simulink library "MOVH"  (R2016a)
settings: Solver=ode45  StartTime=0.0  StopTime=10.0  RelTol=1e-3
undefined symbols (not defined in the file): ALLOWED_ERROR_VALUE, BACKWARD, CCW, CW, FORWARD, MOVE_TURN_LEFT, MOVE_TURN_RIGHT, MOVE_U_TURN, MOVE_U_TURN_LEFT, MOVE_U_TURN_RIGHT, NO_ERROR, ROB_EAST, ROB_NORTH, ROB_SOUTH, ROB_WEST, STOP
libraries: simulink x2
settings Model: Creator=oelkawok  LastModifiedBy=oelkawok
settings DataIOCC: LimitDataPoints=on
settings DebuggingCC: AllowSymbolicDim=off

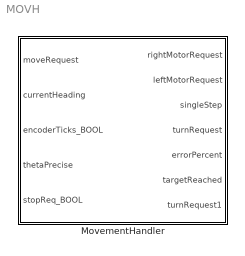
== system MOVH ==
  MovementHandler : Subsystem

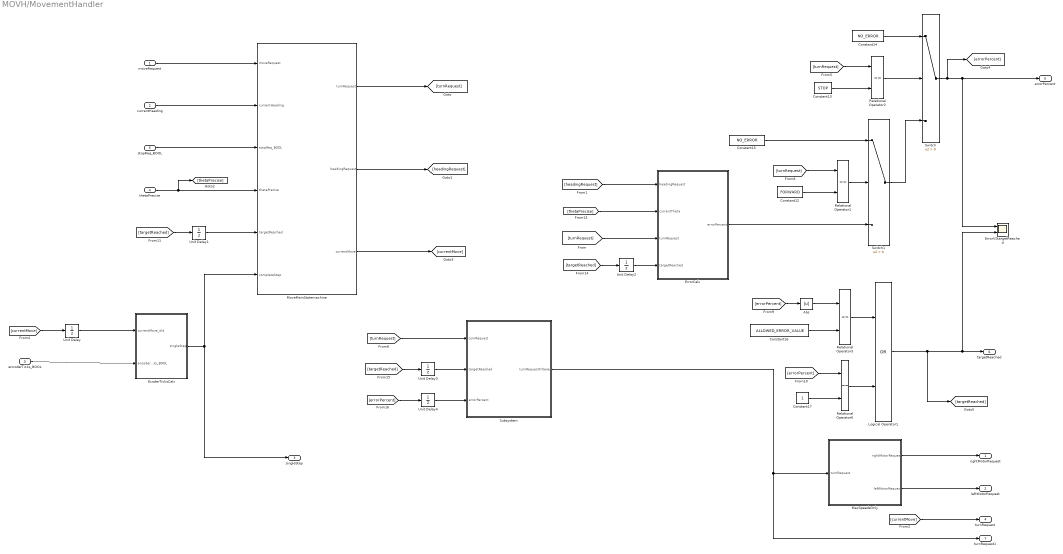
== system MOVH/MovementHandler ==
  moveRequest : Inport
  currentHeading : Inport  Port=2
  encoderTicks_BOOL : Inport  Port=3  PortDimensions=1
  thetaPrecise : Inport  Port=4  PortDimensions=1
  stopReq_BOOL : Inport  Port=5  PortDimensions=1
  Abs : Abs
  Constant12 : Constant  Value=FORWARD
  Constant13 : Constant  Value=STOP
  Constant14 : Constant  Value=NO_ERROR
  Constant15 : Constant  Value=NO_ERROR
  Constant16 : Constant  Value=ALLOWED_ERROR_VALUE
  Constant17 : Constant
  EcoderTicksCalc : Subsystem
  ErrorCalc : Subsystem
  ErrorVStargetReached : Scope  NumInputPorts=2
  Logical Operator1 : Logic  Operator=OR  AllPortsSameDT=off  OutDataTypeStr=boolean
  MaxSpeedsOnly : Subsystem
  MoveMainStatemachine : Subsystem
  Relational Operator1 : RelationalOperator  Operator===  OutDataTypeStr=boolean
  Relational Operator2 : RelationalOperator  Operator===  OutDataTypeStr=boolean
  Relational Operator3 : RelationalOperator  Operator=<=  OutDataTypeStr=boolean
  Relational Operator6 : RelationalOperator  Operator===  OutDataTypeStr=boolean
  Subsystem : Subsystem
  Switch : Switch  Criteria=u2 > Threshold
  Switch1 : Switch  Criteria=u2 > Threshold
  Unit Delay : UnitDelay  InitialCondition=STOP  SampleTime=-1
      settings: AttributesFormatString=%<InitialCondition>
  Unit Delay{1..4} (4 alike) : UnitDelay  InitialCondition=NO_ERROR  SampleTime=-1
      settings: AttributesFormatString=%<InitialCondition>
  rightMotorRequest : Outport
  leftMotorRequest : Outport  Port=2
  singleStep : Outport  Port=3
  turnRequest : Outport  Port=4
  errorPercent : Outport  Port=5  OutputWhenDisabled=reset  InitialOutput=0
  targetReached : Outport  Port=6  OutputWhenDisabled=reset  InitialOutput=0
  turnRequest1 : Outport  Port=7
  wires:
  encoderTicks_BOOL/1 -> EcoderTicksCalc/2(encoderTicks_BOOL)
  EcoderTicksCalc/1(singleStep) -> singleStep/1, MoveMainStatemachine/6(completeStep)
  Constant15/1 -> Switch1/1
  Subsystem/1(turnRequestFiltered) -> turnRequest1/1, MaxSpeedsOnly/1(turnRequest)
  Abs/1 -> Relational Operator3/1
  [errorPercent] -> Unit Delay4/1
  Unit Delay4/1 -> Subsystem/3(errorPercent)
  Unit Delay3/1 -> Subsystem/2(targetReached)
  [targetReached] -> Unit Delay3/1
  Unit Delay2/1 -> ErrorCalc/4(targetReached)
  [targetReached] -> Unit Delay2/1
  Logical Operator1/1 -> targetReached/1, ErrorVStargetReached/2, [targetReached]
  Relational Operator6/1 -> Logical Operator1/2
  Relational Operator3/1 -> Logical Operator1/1
  Constant17/1 -> Relational Operator6/2
  [errorPercent] -> Relational Operator6/1
  Constant16/1 -> Relational Operator3/2
  [errorPercent] -> Abs/1
  Switch/1 -> errorPercent/1, ErrorVStargetReached/1, [errorPercent]
  ErrorCalc/1(errorPercent) -> Switch1/3
  Relational Operator1/1 -> Switch1/2
  [turnRequest] -> Relational Operator1/1
  Constant12/1 -> Relational Operator1/2
  Switch1/1 -> Switch/3
  Constant14/1 -> Switch/1
  Relational Operator2/1 -> Switch/2
  [turnRequest] -> Relational Operator2/1
  Constant13/1 -> Relational Operator2/2
  [currentMove] -> turnRequest/1
  [turnRequest] -> ErrorCalc/3(turnRequest)
  [headingRequest] -> ErrorCalc/1(headingRequest)
  [turnRequest] -> Subsystem/1(turnRequest)
  MaxSpeedsOnly/2(leftMotorRequest) -> leftMotorRequest/1
  MaxSpeedsOnly/1(rightMotorRequest) -> rightMotorRequest/1
  [currentMove] -> Unit Delay/1
  moveRequest/1 -> MoveMainStatemachine/1(moveRequest)
  stopReq_BOOL/1 -> MoveMainStatemachine/3(stopReq_BOOL)
  MoveMainStatemachine/1(turnRequest) -> [turnRequest]
  MoveMainStatemachine/2(headingRequest) -> [headingRequest]
  MoveMainStatemachine/3(currentMove) -> [currentMove]
  currentHeading/1 -> MoveMainStatemachine/2(currentHeading)
  thetaPrecise/1 -> [thetaPrecise], MoveMainStatemachine/4(thetaPrecise)
  [thetaPrecise] -> ErrorCalc/2(currentTheta)
  [targetReached] -> Unit Delay1/1
  Unit Delay1/1 -> MoveMainStatemachine/5(targetReached)
  Unit Delay/1 -> EcoderTicksCalc/1(currentMove_old)

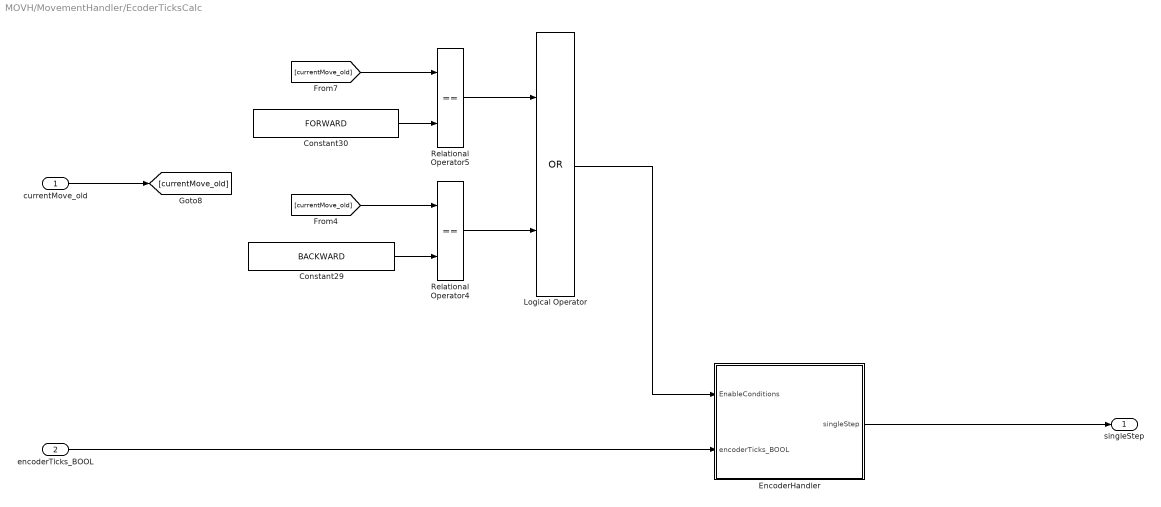
== system MOVH/MovementHandler/EcoderTicksCalc ==
  currentMove_old : Inport
  encoderTicks_BOOL : Inport  Port=2
  Constant29 : Constant  Value=BACKWARD
  Constant30 : Constant  Value=FORWARD
  EncoderHandler : Subsystem
  Logical Operator : Logic  Operator=OR  AllPortsSameDT=off  OutDataTypeStr=boolean
  Relational Operator4 : RelationalOperator  Operator===  OutDataTypeStr=boolean
  Relational Operator5 : RelationalOperator  Operator===  OutDataTypeStr=boolean
  singleStep : Outport
  wires:
  currentMove_old/1 -> [currentMove_old]
  EncoderHandler/1(singleStep) -> singleStep/1
  Relational Operator4/1 -> Logical Operator/2
  Relational Operator5/1 -> Logical Operator/1
  [currentMove_old] -> Relational Operator5/1
  Constant30/1 -> Relational Operator5/2
  [currentMove_old] -> Relational Operator4/1
  Logical Operator/1 -> EncoderHandler/1(EnableConditions)
  encoderTicks_BOOL/1 -> EncoderHandler/2(encoderTicks_BOOL)
  Constant29/1 -> Relational Operator4/2

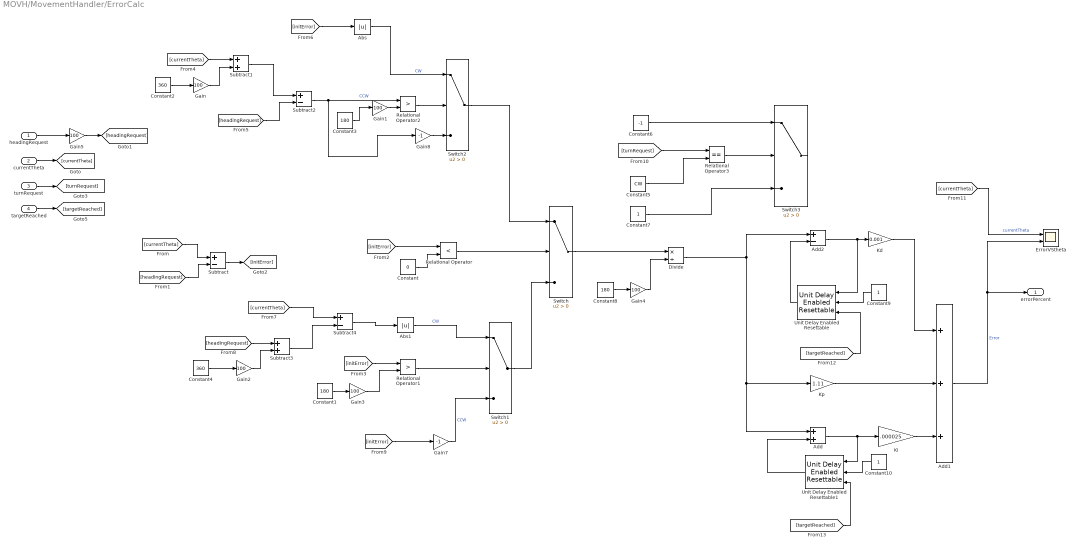
== system MOVH/MovementHandler/ErrorCalc ==
  headingRequest : Inport
  currentTheta : Inport  Port=2
  turnRequest : Inport  Port=3
  targetReached : Inport  Port=4
  Abs : Abs
  Abs1 : Abs
  Add : Sum
  Add1 : Sum  Inputs=+++
  Add2 : Sum  Inputs=+-
  Constant : Constant  Value=0
  Constant1 : Constant  Value=180
  Constant10 : Constant
  Constant2 : Constant  Value=360
  Constant3 : Constant  Value=180
  Constant4 : Constant  Value=360
  Constant5 : Constant  Value=CW
  Constant6 : Constant  Value=-1
  Constant7 : Constant
  Constant8 : Constant  Value=180
  Constant9 : Constant
  Divide : Product  Inputs=*/
  ErrorVStheta : Scope  NumInputPorts=2
  Gain{,1..5} (6 alike) : Gain  Gain=100
  Gain7 : Gain  Gain=-1
  Gain8 : Gain  Gain=-1
  Kd : Gain  Gain=0.001
  Ki : Gain  Gain=.000025
  Kp : Gain  Gain=1.11
  Relational Operator : RelationalOperator  Operator=<  OutDataTypeStr=boolean
  Relational Operator1 : RelationalOperator  Operator=>  OutDataTypeStr=boolean
  Relational Operator2 : RelationalOperator  Operator=>  OutDataTypeStr=boolean
  Relational Operator3 : RelationalOperator  Operator===  OutDataTypeStr=boolean
  Subtract : Sum  Inputs=+-
  Subtract1 : Sum
  Subtract2 : Sum  Inputs=+-
  Subtract3 : Sum
  Subtract4 : Sum  Inputs=+-
  Switch{,1..3} (4 alike) : Switch  Criteria=u2 > Threshold
  Unit Delay Enabled Resettable : simulink/Additional Math & Discrete/Additional Discrete/Unit Delay Enabled Resettable  vinit=0.0  tsamp=-1
  Unit Delay Enabled Resettable1 : simulink/Additional Math & Discrete/Additional Discrete/Unit Delay Enabled Resettable  vinit=0.0  tsamp=-1
  errorPercent : Outport  OutputWhenDisabled=reset  InitialOutput=0
  wires:
  Gain8/1 -> Switch2/3
  Gain7/1 -> Switch1/3  "CCW"
  [targetReached] -> Unit Delay Enabled Resettable1/3
  Constant10/1 -> Unit Delay Enabled Resettable1/2
  [targetReached] -> Unit Delay Enabled Resettable/3
  targetReached/1 -> [targetReached]
  Constant9/1 -> Unit Delay Enabled Resettable/2
  Gain5/1 -> [headingRequest]
  Gain4/1 -> Divide/2
  Gain3/1 -> Relational Operator1/2
  Gain2/1 -> Subtract3/2
  Gain1/1 -> Relational Operator2/2
  Gain/1 -> Subtract1/2
  [currentTheta] -> ErrorVStheta/1  "currentTheta"
  Add1/1 -> errorPercent/1, ErrorVStheta/2  "Error"
  Kp/1 -> Add1/2
  Kd/1 -> Add1/1
  Unit Delay Enabled Resettable/1 -> Add2/2
  Add2/1 -> Kd/1, Unit Delay Enabled Resettable/1
  Ki/1 -> Add1/3
  Unit Delay Enabled Resettable1/1 -> Add/2
  Add/1 -> Ki/1, Unit Delay Enabled Resettable1/1
  Divide/1 -> Add/1, Kp/1, Add2/1
  Constant/1 -> Relational Operator/2
  Relational Operator/1 -> Switch/2
  Relational Operator1/1 -> Switch1/2
  Constant1/1 -> Gain3/1
  Switch1/1 -> Switch/3
  headingRequest/1 -> Gain5/1
  currentTheta/1 -> [currentTheta]
  [headingRequest] -> Subtract/2
  [currentTheta] -> Subtract/1
  Subtract/1 -> [initError]
  [initError] -> Relational Operator/1
  [initError] -> Relational Operator1/1
  [currentTheta] -> Subtract1/1
  Constant2/1 -> Gain/1
  Subtract1/1 -> Subtract2/1
  [headingRequest] -> Subtract2/2
  Constant3/1 -> Gain1/1
  Subtract2/1 -> Relational Operator2/1, Gain8/1  "CCW"
  Relational Operator2/1 -> Switch2/2
  Switch2/1 -> Switch/1
  [initError] -> Abs/1
  Abs/1 -> Switch2/1  "CW"
  Constant4/1 -> Gain2/1
  [headingRequest] -> Subtract3/1
  [currentTheta] -> Subtract4/1
  Subtract3/1 -> Subtract4/2
  Subtract4/1 -> Abs1/1
  Abs1/1 -> Switch1/1  "CW"
  [initError] -> Gain7/1
  turnRequest/1 -> [turnRequest]
  [turnRequest] -> Relational Operator3/1
  Constant5/1 -> Relational Operator3/2
  Relational Operator3/1 -> Switch3/2
  Constant6/1 -> Switch3/1
  Constant7/1 -> Switch3/3
  Switch/1 -> Divide/1
  Constant8/1 -> Gain4/1

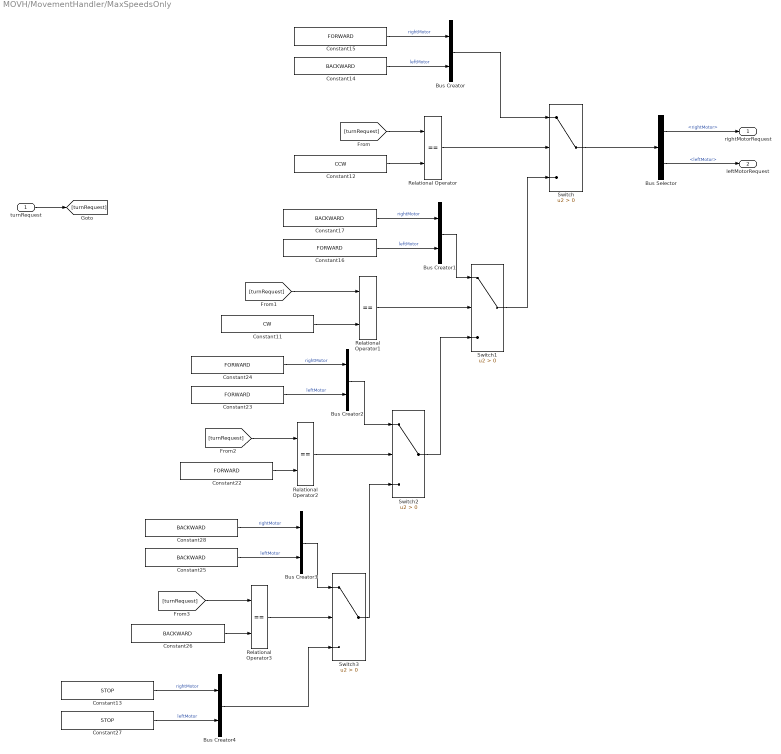
== system MOVH/MovementHandler/MaxSpeedsOnly ==
  turnRequest : Inport
  Bus Creator{,1..4} (5 alike) : BusCreator  Inputs=2
  Bus Selector : BusSelector  OutputSignals=rightMotor,leftMotor
  Constant11 : Constant  Value=CW
  Constant12 : Constant  Value=CCW
  Constant13 : Constant  Value=STOP
  Constant{14,17,25..26,28} (5 alike) : Constant  Value=BACKWARD
  Constant{15..16,22..24} (5 alike) : Constant  Value=FORWARD
  Constant27 : Constant  Value=STOP
  Relational Operator{,1..3} (4 alike) : RelationalOperator  Operator===  OutDataTypeStr=boolean
  Switch{,1..3} (4 alike) : Switch  Criteria=u2 > Threshold
  rightMotorRequest : Outport
  leftMotorRequest : Outport  Port=2
  wires:
  turnRequest/1 -> [turnRequest]
  Constant13/1 -> Bus Creator4/1  "rightMotor"
  Constant23/1 -> Bus Creator2/2  "leftMotor"
  Bus Creator3/1 -> Switch3/1
  Constant27/1 -> Bus Creator4/2  "leftMotor"
  Switch3/1 -> Switch2/3
  Bus Creator4/1 -> Switch3/3
  Bus Creator2/1 -> Switch2/1
  Constant26/1 -> Relational Operator3/2
  Constant25/1 -> Bus Creator3/2  "leftMotor"
  Constant28/1 -> Bus Creator3/1  "rightMotor"
  Relational Operator2/1 -> Switch2/2
  Switch2/1 -> Switch1/3
  Constant22/1 -> Relational Operator2/2
  [turnRequest] -> Relational Operator2/1
  Relational Operator3/1 -> Switch3/2
  Relational Operator1/1 -> Switch1/2
  Constant24/1 -> Bus Creator2/1  "rightMotor"
  Constant11/1 -> Relational Operator1/2
  Bus Creator1/1 -> Switch1/1
  Constant17/1 -> Bus Creator1/1  "rightMotor"
  [turnRequest] -> Relational Operator3/1
  Switch1/1 -> Switch/3
  Bus Selector/2 -> leftMotorRequest/1  "<leftMotor>"
  Constant16/1 -> Bus Creator1/2  "leftMotor"
  Bus Selector/1 -> rightMotorRequest/1  "<rightMotor>"
  [turnRequest] -> Relational Operator1/1
  Bus Creator/1 -> Switch/1
  Constant14/1 -> Bus Creator/2  "leftMotor"
  Switch/1 -> Bus Selector/1
  [turnRequest] -> Relational Operator/1
  Relational Operator/1 -> Switch/2
  Constant12/1 -> Relational Operator/2
  Constant15/1 -> Bus Creator/1  "rightMotor"

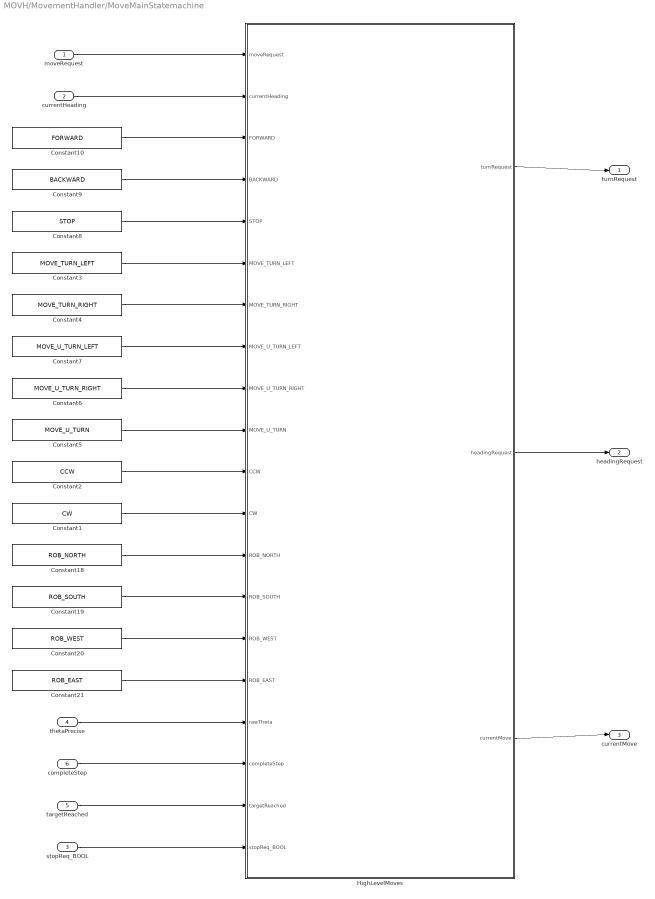
== system MOVH/MovementHandler/MoveMainStatemachine ==
  moveRequest : Inport
  currentHeading : Inport  Port=2
  stopReq_BOOL : Inport  Port=3  PortDimensions=1
  thetaPrecise : Inport  Port=4  PortDimensions=1
  targetReached : Inport  Port=5  PortDimensions=1
  completeStep : Inport  Port=6  PortDimensions=1
  Constant1 : Constant  Value=CW
  Constant10 : Constant  Value=FORWARD
  Constant18 : Constant  Value=ROB_NORTH
  Constant19 : Constant  Value=ROB_SOUTH
  Constant2 : Constant  Value=CCW
  Constant20 : Constant  Value=ROB_WEST
  Constant21 : Constant  Value=ROB_EAST
  Constant3 : Constant  Value=MOVE_TURN_LEFT
  Constant4 : Constant  Value=MOVE_TURN_RIGHT
  Constant5 : Constant  Value=MOVE_U_TURN
  Constant6 : Constant  Value=MOVE_U_TURN_RIGHT
  Constant7 : Constant  Value=MOVE_U_TURN_LEFT
  Constant8 : Constant  Value=STOP
  Constant9 : Constant  Value=BACKWARD
  HighLevelMoves : Stateflow chart  TreatAsAtomicUnit=on
  turnRequest : Outport
  headingRequest : Outport  Port=2
  currentMove : Outport  Port=3
  wires:
  stopReq_BOOL/1 -> HighLevelMoves/20(stopReq_BOOL)
  Constant5/1 -> HighLevelMoves/10(MOVE_U_TURN)
  Constant21/1 -> HighLevelMoves/16(ROB_EAST)
  Constant2/1 -> HighLevelMoves/11(CCW)
  Constant18/1 -> HighLevelMoves/13(ROB_NORTH)
  Constant19/1 -> HighLevelMoves/14(ROB_SOUTH)
  Constant20/1 -> HighLevelMoves/15(ROB_WEST)
  HighLevelMoves/2(headingRequest) -> headingRequest/1
  moveRequest/1 -> HighLevelMoves/1(moveRequest)
  currentHeading/1 -> HighLevelMoves/2(currentHeading)
  Constant4/1 -> HighLevelMoves/7(MOVE_TURN_RIGHT)
  HighLevelMoves/3(currentMove) -> currentMove/1
  HighLevelMoves/1(turnRequest) -> turnRequest/1
  Constant8/1 -> HighLevelMoves/5(STOP)
  Constant10/1 -> HighLevelMoves/3(FORWARD)
  Constant9/1 -> HighLevelMoves/4(BACKWARD)
  Constant3/1 -> HighLevelMoves/6(MOVE_TURN_LEFT)
  Constant7/1 -> HighLevelMoves/8(MOVE_U_TURN_LEFT)
  Constant6/1 -> HighLevelMoves/9(MOVE_U_TURN_RIGHT)
  Constant1/1 -> HighLevelMoves/12(CW)
  completeStep/1 -> HighLevelMoves/18(completeStep)
  thetaPrecise/1 -> HighLevelMoves/17(rawTheta)
  targetReached/1 -> HighLevelMoves/19(targetReached)

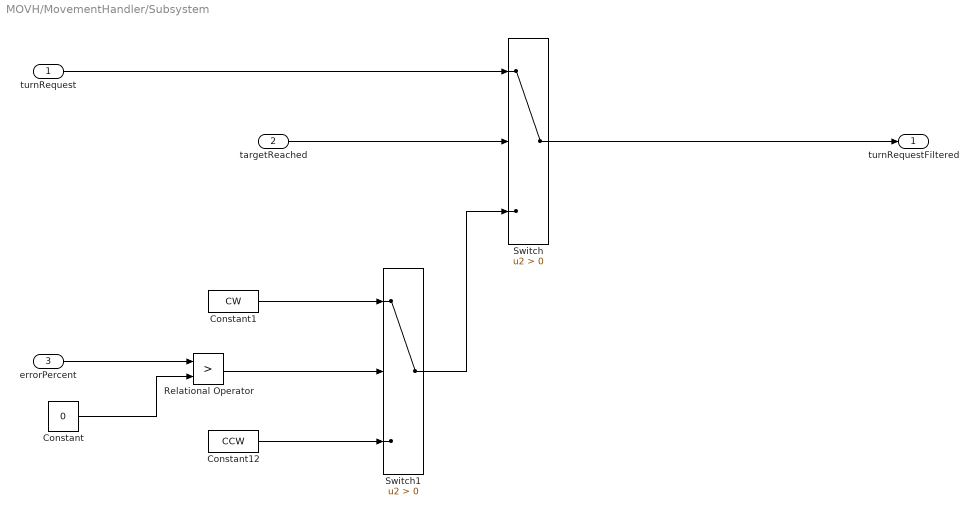
== system MOVH/MovementHandler/Subsystem ==
  turnRequest : Inport
  targetReached : Inport  Port=2
  errorPercent : Inport  Port=3
  Constant : Constant  Value=0
  Constant1 : Constant  Value=CW
  Constant12 : Constant  Value=CCW
  Relational Operator : RelationalOperator  Operator=>  OutDataTypeStr=boolean
  Switch : Switch  Criteria=u2 > Threshold
  Switch1 : Switch  Criteria=u2 > Threshold
  turnRequestFiltered : Outport
  wires:
  Constant1/1 -> Switch1/1
  Constant12/1 -> Switch1/3
  Switch/1 -> turnRequestFiltered/1
  turnRequest/1 -> Switch/1
  Constant/1 -> Relational Operator/2
  errorPercent/1 -> Relational Operator/1
  Relational Operator/1 -> Switch1/2
  Switch1/1 -> Switch/3
  targetReached/1 -> Switch/2

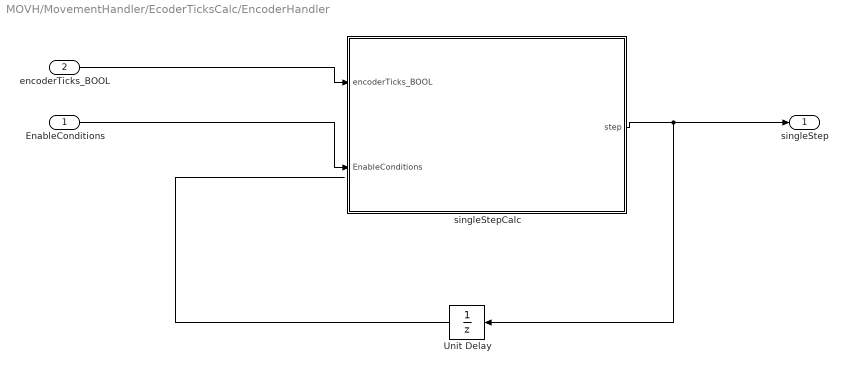
== system MOVH/MovementHandler/EcoderTicksCalc/EncoderHandler ==
  EnableConditions : Inport  PortDimensions=1
  encoderTicks_BOOL : Inport  Port=2  PortDimensions=1
  Unit Delay : UnitDelay  SampleTime=-1
  singleStepCalc : Stateflow chart  TreatAsAtomicUnit=on
  singleStep : Outport  OutputWhenDisabled=reset  InitialOutput=0
  wires:
  EnableConditions/1 -> singleStepCalc/2(EnableConditions)
  Unit Delay/1 -> ?
  encoderTicks_BOOL/1 -> singleStepCalc/1(encoderTicks_BOOL)
  singleStepCalc/1(step) -> singleStep/1, Unit Delay/1

== stateflow chart MOVH/MovementHandler/EcoderTicksCalc/EncoderHandler/singleStepCalc ==
  state Running
    state PosEdge
      entry:
      counter++;
    state High
    state step
      entry:
      step = true;
      counter = 0;
    (default) -> High
    High -> PosEdge : [hasChanged(encoderTicks_BOOL)...
        | && encoderTicks_BOOL == true]
        | /step = false;
    PosEdge -> High [order 2]
    step -> High
    PosEdge -> step [order 1] : [counter >= 35]
  state Idle
    state Rise
      en:
      step = true;
    state Idle
      en:
      step = false;
    (default) -> (junction 23)
    (junction 23) -> Rise [order 1] : [counter >= (35*0.75)]
    (junction 23) -> Idle.Idle [order 2]
  state Init
    entry:
    counter = 0;
  (default) -> Init
  Init -> Running
  Running -> Idle : [EnableConditions == false]
      | /step = false;
  Idle -> Running : [EnableConditions == true]
      | /step = false;
      | counter = 0;
  data: encoderTicks_BOOL input; step output boolean; counter local uint16; EnableConditions input

== stateflow chart MOVH/MovementHandler/MoveMainStatemachine/HighLevelMoves ==
  state Stop
  state forward
    state fixingHeading
    state Idle
    (junction 252) -> fixingHeading [order 1] : [(rawTheta < 90*100)...
        | || (rawTheta > 270*100)]
        | /turnRequest = CCW;
    (default) -> Idle
    (junction 252) -> fixingHeading [order 2] : /turnRequest = CW;
    (junction 250) -> (junction 252) [order 1] : [headingRequest == ROB_NORTH]
    (junction 253) -> fixingHeading [order 1] : [(rawTheta < 90*100)...
        | || (rawTheta > 270*100)]
        | /turnRequest = CW;
    (junction 250) -> (junction 253) [order 2] : [headingRequest == ROB_SOUTH]
    (junction 253) -> fixingHeading [order 2] : /turnRequest = CCW;
    Idle -> (junction 270)
    (junction 270) -> (junction 250) [order 1] : [!((rawTheta >= (headingRequest*100) - 100)...
        | && (rawTheta <= (headingRequest*100) + 100))]
    (junction 250) -> (junction 254) [order 3] : [headingRequest == ROB_EAST]
    (junction 270) -> Idle [order 2] : [(rawTheta >= (headingRequest*100) - 100)...
        | && (rawTheta <= (headingRequest*100) + 100)]
        | /turnRequest = FORWARD;
    (junction 250) -> (junction 255) [order 4] : [headingRequest == ROB_WEST]
    (junction 254) -> fixingHeading [order 1] : [rawTheta > 180*100]
        | /turnRequest = CW;
    (junction 254) -> fixingHeading [order 2] : /turnRequest = CCW;
    (junction 255) -> fixingHeading [order 1] : [rawTheta > 180*100]
        | /turnRequest = CCW;
    fixingHeading -> Idle
    (junction 255) -> fixingHeading [order 2] : /turnRequest = CW;
  state TurnLeft
    state finish
      entry:
      turnActive = false;
    state start
      entry:
      turnRequest = CCW;
      turnActive = true;
    state turning
    (default) -> TurnLeft.start
    TurnLeft.start -> TurnLeft.turning [order 1] : [currentHeading == ROB_NORTH]
        | /headingRequest = ROB_WEST;
    TurnLeft.start -> TurnLeft.turning [order 3] : [currentHeading == ROB_SOUTH]
        | /headingRequest = ROB_EAST;
    TurnLeft.turning -> TurnLeft.finish : [(currentHeading == headingRequest)...
        | && (targetReached == true)]
    TurnLeft.start -> TurnLeft.turning [order 4] : [currentHeading == ROB_WEST]
        | /headingRequest = ROB_SOUTH;
    TurnLeft.start -> TurnLeft.turning [order 2] : [currentHeading == ROB_EAST]
        | /headingRequest = ROB_NORTH;
  state backward
  state UturnLeft
    entry:
    uTurnCounter = 0;
    state finish
      entry:
      turnActive = false;
    state TurnLeft
      state finish
        entry:
        uTurnCounter = uTurnCounter + 1;
      state start
        entry:
        turnRequest = CCW;
        turnActive = true;
      state turning
      (default) -> UturnLeft.TurnLeft.start
      UturnLeft.TurnLeft.start -> UturnLeft.TurnLeft.turning [order 1] : [currentHeading == ROB_NORTH]
          | /headingRequest = ROB_WEST;
      UturnLeft.TurnLeft.start -> UturnLeft.TurnLeft.turning [order 3] : [currentHeading == ROB_SOUTH]
          | /headingRequest = ROB_EAST;
      UturnLeft.TurnLeft.turning -> UturnLeft.TurnLeft.finish : [(currentHeading == headingRequest)...
          | && (targetReached == true)]
      UturnLeft.TurnLeft.start -> UturnLeft.TurnLeft.turning [order 4] : [currentHeading == ROB_WEST]
          | /headingRequest = ROB_SOUTH;
      UturnLeft.TurnLeft.start -> UturnLeft.TurnLeft.turning [order 2] : [currentHeading == ROB_EAST]
          | /headingRequest = ROB_NORTH;
    state forwardStep
      entry:
      counter = 0;
      turnRequest = FORWARD;
      currentMove = FORWARD;
      du:
      counter++;
    (default) -> UturnLeft.TurnLeft
    UturnLeft.TurnLeft -> UturnLeft.finish [order 2] : [uTurnCounter == 2]
    UturnLeft.TurnLeft -> UturnLeft.forwardStep [order 1] : [(uTurnCounter == 1)...
        | && hasChanged(uTurnCounter)]
    UturnLeft.forwardStep -> UturnLeft.TurnLeft [order 1] : [((counter >= 2)...
        | && moveDone == true)...
        | || (stopReq_BOOL == true)]
        | /moveDone = false;
        | currentMove = MOVE_U_TURN_LEFT;
    UturnLeft.forwardStep -> UturnLeft.forwardStep [order 2] : [(hasChanged(completeStep))...
        | && (completeStep == true)]
        | /moveDone = true;
  state Uturn
    entry:
    uTurnCounter = 0;
    state finish
      entry:
      turnActive = false;
    state TurnRight
      state finish
        uTurnCounter = uTurnCounter + 1;
      state turning
      state start
        entry:
        turnRequest = CW;
        turnActive = true;
      (default) -> Uturn.TurnRight.start
      Uturn.TurnRight.start -> Uturn.TurnRight.turning [order 2] : [currentHeading == ROB_NORTH]
          | /headingRequest = ROB_EAST;
      Uturn.TurnRight.start -> Uturn.TurnRight.turning [order 4] : [currentHeading == ROB_SOUTH]
          | /headingRequest = ROB_WEST;
      Uturn.TurnRight.turning -> Uturn.TurnRight.finish : [(currentHeading == headingRequest)...
          | && (targetReached == true)]
      Uturn.TurnRight.start -> Uturn.TurnRight.turning [order 3] : [currentHeading == ROB_WEST]
          | /headingRequest = ROB_NORTH;
      Uturn.TurnRight.start -> Uturn.TurnRight.turning [order 1] : [currentHeading == ROB_EAST]
          | /headingRequest = ROB_SOUTH;
    Uturn.TurnRight -> Uturn.TurnRight [order 1] : [(uTurnCounter == 1)...
        | && hasChanged(uTurnCounter)]
    (default) -> Uturn.TurnRight
    Uturn.TurnRight -> Uturn.finish [order 2] : [uTurnCounter == 2]
  state TurnRight
    state turning
    state finish
      entry:
      turnActive = false;
    state start
      entry:
      turnRequest = CW;
      turnActive = true;
    (default) -> TurnRight.start
    TurnRight.start -> TurnRight.turning [order 2] : [currentHeading == ROB_NORTH]
        | /headingRequest = ROB_EAST;
    TurnRight.start -> TurnRight.turning [order 4] : [currentHeading == ROB_SOUTH]
        | /headingRequest = ROB_WEST;
    TurnRight.turning -> TurnRight.finish : [(currentHeading == headingRequest)...
        | && (targetReached == true)]
    TurnRight.start -> TurnRight.turning [order 3] : [currentHeading == ROB_WEST]
        | /headingRequest = ROB_NORTH;
    TurnRight.start -> TurnRight.turning [order 1] : [currentHeading == ROB_EAST]
        | /headingRequest = ROB_SOUTH;
  state UturnRight
    entry:
    uTurnCounter = 0;
    state finish
      entry:
      turnActive = false;
    state TurnRight
      state start
        entry:
        turnRequest = CW;
        turnActive = true;
      state finish
        entry:
        uTurnCounter = uTurnCounter + 1;
      state turning
      (default) -> UturnRight.TurnRight.start
      UturnRight.TurnRight.start -> UturnRight.TurnRight.turning [order 2] : [currentHeading == ROB_NORTH]
          | /headingRequest = ROB_EAST;
      UturnRight.TurnRight.start -> UturnRight.TurnRight.turning [order 4] : [currentHeading == ROB_SOUTH]
          | /headingRequest = ROB_WEST;
      UturnRight.TurnRight.turning -> UturnRight.TurnRight.finish : [(currentHeading...
          |  == headingRequest)...
          | && (targetReached == true)]
      UturnRight.TurnRight.start -> UturnRight.TurnRight.turning [order 3] : [currentHeading == ROB_WEST]
          | /headingRequest = ROB_NORTH;
      UturnRight.TurnRight.start -> UturnRight.TurnRight.turning [order 1] : [currentHeading == ROB_EAST]
          | /headingRequest = ROB_SOUTH;
    state forwardStep
      entry:
      counter = 0;
      turnRequest = FORWARD;
      currentMove = FORWARD;
      du:
      counter++;
    (default) -> UturnRight.TurnRight
    UturnRight.TurnRight -> UturnRight.finish [order 2] : [uTurnCounter == 2]
    UturnRight.TurnRight -> UturnRight.forwardStep [order 1] : [hasChanged(uTurnCounter) ...
        | && (uTurnCounter == 1)]
    UturnRight.forwardStep -> UturnRight.TurnRight [order 1] : [((counter >= 2)...
        | && moveDone == true)...
        | || (stopReq_BOOL == true)]
        | /moveDone = false;
        | currentMove = MOVE_U_TURN_RIGHT;
    UturnRight.forwardStep -> UturnRight.forwardStep [order 2] : [(hasChanged(completeStep))...
        | && (completeStep == true)]
        | /moveDone = true;
  (default) -> Stop : /headingRequest = ROB_NORTH;
  Stop -> (junction 9) : [hasChanged(moveRequest) ...
      | || (turnActive == false)]
  (junction 9) -> Stop [order 6] : [moveRequest == STOP]
      | /turnRequest = STOP;
      | currentMove = STOP;
  forward -> (junction 9) : [hasChanged(moveRequest)]
  (junction 9) -> TurnLeft [order 8] : [(moveRequest == MOVE_TURN_LEFT)]
      | /currentMove = MOVE_TURN_LEFT;
  (junction 9) -> forward [order 1] : [moveRequest == FORWARD]
      | /turnRequest = FORWARD;
      | currentMove = FORWARD;
  TurnLeft -> (junction 9) : [hasChanged(moveRequest) ...
      | || (turnActive == false)]
  (junction 9) -> backward [order 2] : [moveRequest == BACKWARD]
      | /turnRequest = BACKWARD;
      | currentMove = BACKWARD;
  (junction 9) -> UturnLeft [order 5] : [(moveRequest == MOVE_U_TURN_LEFT)]
      | /currentMove = MOVE_U_TURN_LEFT;
  backward -> (junction 9) : [hasChanged(moveRequest) ...
      | || (turnActive == false)]
  Uturn -> (junction 9) : [hasChanged(moveRequest) ...
      | || (turnActive == false)]
  UturnLeft -> (junction 9) : [hasChanged(moveRequest) ...
      | || (turnActive == false)]
  (junction 9) -> TurnRight [order 7] : [(moveRequest == MOVE_TURN_RIGHT)]
      | /currentMove = MOVE_TURN_RIGHT;
  (junction 9) -> Uturn [order 4] : [moveRequest == MOVE_U_TURN]
      | /currentMove = MOVE_U_TURN;
  UturnRight -> (junction 9) : [hasChanged(moveRequest) ...
      | || (turnActive == false)]
  TurnRight -> (junction 9) : [hasChanged(moveRequest) ...
      | || (turnActive == false)]
  (junction 9) -> UturnRight [order 3] : [(moveRequest == MOVE_U_TURN_RIGHT)]
      | /currentMove = MOVE_U_TURN_RIGHT;
  data: moveRequest input; currentHeading input; FORWARD input; BACKWARD input; STOP input; MOVE_TURN_LEFT input; MOVE_TURN_RIGHT input; MOVE_U_TURN_LEFT input; MOVE_U_TURN_RIGHT input; MOVE_U_TURN input; turnRequest output double; headingRequest output double; CCW input double; CW input double; ROB_NORTH input; ROB_SOUTH input; ROB_WEST input; ROB_EAST input; rawTheta input; turnActive local double; completeStep input; uTurnCounter local double; counter local double; moveDone local double; currentMove output double; targetReached input; stopReq_BOOL input
